simulink model "SemiOffline_Preprocessing_SCG3D"  (R2019a)
settings: Solver=FixedStepDiscrete  StartTime=0.0  StopTime=2*sim_time  FixedStep=1/fs  MaxStep=1/fs  RelTol=1e-3
undefined symbols (not defined in the file): fdesignblkfcn, fs, gcbh, tot_samples
settings Model: Creator=rcord  LastModifiedBy=rcord
settings DataIOCC: ExternalInput=[t, x, y, z]  LoadExternalInput=on
settings DebuggingCC: UnderSpecifiedDimensionMsg=warning

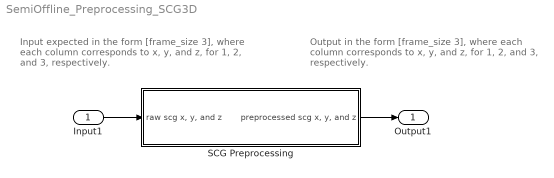
== system SemiOffline_Preprocessing_SCG3D ==
  note: Input expected in the form [frame_size 3],
      | where each column corresponds to x, y, and z,
      | for 1, 2, and 3, respectively.
  note: Output in the form [frame_size 3],
      | where each column corresponds to x, y, and z,
      | for 1, 2, and 3, respectively.
  Input1 : Inport  SampleTime=1/fs
  SCG Preprocessing : Subsystem  mask{param_scg_gain_mg=3333, param_scg_fc_lo=5, param_scg_fc_hi=40, param_scg_trans_bw=2.5}
      mask prompts: param_scg_gain_mg "V to mg Conversion Gain"; param_scg_fc_lo "Low Passband Frequency Corner (Hz)"; param_scg_fc_hi "High Passband Frequency Corner (Hz)"; param_scg_trans_bw "Transition bandwidth"
      mask init:
      | assignin('base','param_scg_gain_mg',param_scg_gain_mg)
      | assignin('base','param_scg_fc_lo',param_scg_fc_lo)
      | assignin('base','param_scg_fc_hi',param_scg_fc_hi)
      | assignin('base','param_scg_trans_bw',param_scg_trans_bw)
      mask DialogControl DescGroupVar Prompt: SCG Preprocessing
      mask DialogControl DescTextVar Prompt: The preprocesing of the three SCG x, y, and z components passed along a single signal input. The preprocessing consists of a amplifcaiton/conversion stage followed by a filtfilt operation (i.e. a front-back zero-phase FIR bandpass filter).
  Output1 : Outport
  wires:
  Input1/1 -> SCG Preprocessing/1("raw scg x, y, and z")
  SCG Preprocessing/1("preprocessed scg x, y, and z") -> Output1/1

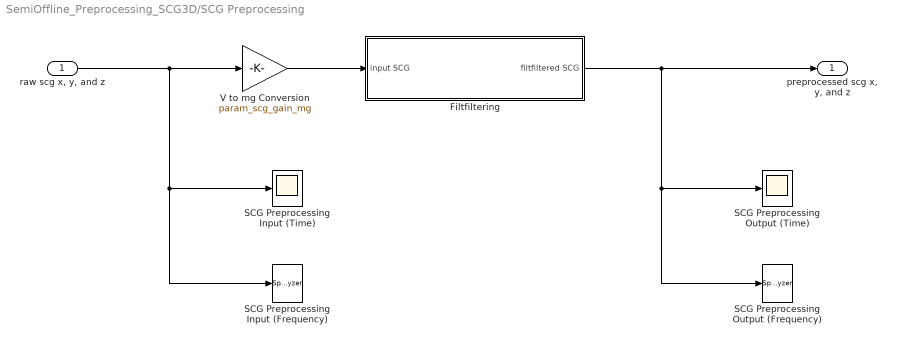
== system SemiOffline_Preprocessing_SCG3D/SCG Preprocessing ==
  "raw scg x, y, and z" : Inport
  Filtfiltering : Subsystem
  SCG Preprocessing Input (Frequency) : SpectrumAnalyzer
  SCG Preprocessing Input (Time) : Scope
  SCG Preprocessing Output (Frequency) : SpectrumAnalyzer
  SCG Preprocessing Output (Time) : Scope
  V to mg Conversion : Gain  Gain=param_scg_gain_mg
  "preprocessed scg x, y, and z" : Outport
  wires:
  V to mg Conversion/1 -> Filtfiltering/1(" input SCG")
  Filtfiltering/1(filtfiltered SCG) -> "preprocessed scg x, y, and z"/1, SCG Preprocessing Output (Frequency)/1, SCG Preprocessing Output (Time)/1
  "raw scg x, y, and z"/1 -> V to mg Conversion/1, SCG Preprocessing Input (Frequency)/1, SCG Preprocessing Input (Time)/1

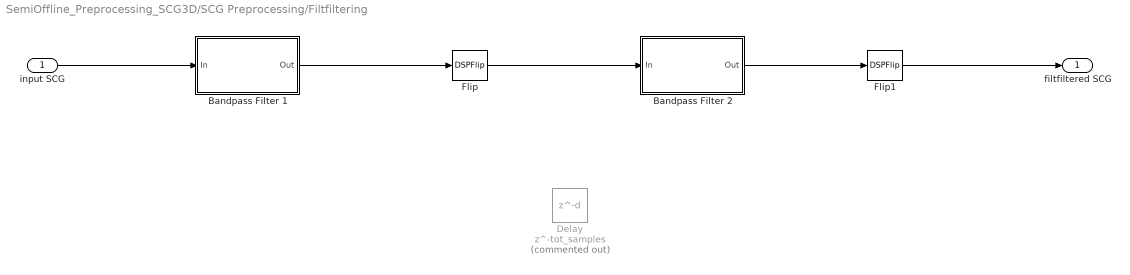
== system SemiOffline_Preprocessing_SCG3D/SCG Preprocessing/Filtfiltering ==
  " input SCG" : Inport
  Bandpass Filter 1 : Subsystem  DialogController=fdesignblkfcn  InitFcn=fdesignblkfcn(gcbh, {'InitFcn'});  mask(Bandpass Filter){}
      mask help: Design a bandpass filter
      settings: CopyFcn=fdesignblkfcn(gcbh, {'CopyFcn'});
      mask Help: helpview(mapfilelocation('dsp'), 'dspbandpassfilter');
      mask Display: disp('Bandpass');
  Bandpass Filter 2 : Subsystem  DialogController=fdesignblkfcn  InitFcn=fdesignblkfcn(gcbh, {'InitFcn'});  mask(Bandpass Filter){}
      mask help: Design a bandpass filter
      settings: CopyFcn=fdesignblkfcn(gcbh, {'CopyFcn'});
      mask Help: helpview(mapfilelocation('dsp'), 'dspbandpassfilter');
      mask Display: disp('Bandpass');
  Delay : Delay  Commented=on  DelayLength=tot_samples
  Flip : DSPFlip
  Flip1 : DSPFlip
  filtfiltered SCG : Outport
  wires:
  Bandpass Filter 2/1(Out) -> Flip1/1
  Bandpass Filter 1/1(Out) -> Flip/1
  Flip1/1 -> filtfiltered SCG/1
  " input SCG"/1 -> Bandpass Filter 1/1(In)
  Flip/1 -> Bandpass Filter 2/1(In)

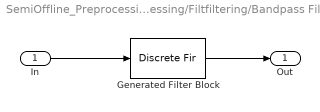
== system SemiOffline_Preprocessing_SCG3D/SCG Preprocessing/Filtfiltering/Bandpass Filter 1 ==
  In : Inport
  Generated Filter Block : DiscreteFir  Tag=BlockMethodSubSystem  Coefficients=[-0.000644776881089011221 -0.000343554860043022352 -0.000418089254709499275 -0.000488742609981019163 -0.000551243345798582566 -0.000600235305924576648 -0.00063171306769246806 -0.000640836865515264807 -0.000623577399542782373 -0.000575229334500284694 -0.000494985950960804763 -0.000381627044804629134 -0.000233865006442936121 -5.56678921839550995e-05 0.000150944750294620727 0.000380332853480295433 0.00062653849699591019 0.000881816649475024436 0.00113740319574445639 0.00138431406995232105 0.00161321911397308633 0.0018146043144366829 0.00198008854337072566 0.00210262259699513969 0.00217572124608666432 0.00219597055848480376 0.00216075573049529434 0.00207097175527305938 0.00192865213177504605 0.00173898123537951027 0.00150863042848189965 0.00124677018487260151 0.000963043907161496653 0.000669179660023357689 0.000376320878595885961 9.62462280283141939e-05 -0.000160563804743702409 -0.000384391646009586794 -0.000567507973019773342 -0.000704030812785294492 -0.00079079232930282504 -0.000826637258703924243 -0.000813548141499978168 -0.000755551211624549946 -0.000659215605623974577 -0.000532703240683185986 -0.000385888389387102669 -0.000229155313949030114 -7.35784921629424322e-05 7.06945997310475362e-05 0.000193741453659791903 0.000287790719150024911 0.000346383593154441817 0.000365847560832936172 0.000344383008930271859 0.000283347463518772609 0.000185853244975725074 5.79335170000474034e-05 -9.32933989238659894e-05 -0.000258576563413746212 -0.0004284890942197088 -0.000592821858813498285 -0.000742242260932749745 -0.00086783910074455324 -0.000962759059241456673 -0.0010215146506733989 -0.00104142267039370319 -0.00102169614249135237 -0.000964510497639283534 -0.000873959783460330681 -0.000756582912594168204 -0.000620183712708287848 -0.000474201473147084441 -0.000328149776762294532 -0.000192029162020909033 -7.46952916294248755e-05 1.57079301373542948e-05 7.32427637147023197e-05 9.36173902064841982e-05 7.54005127585129936e-05 1.91161807097391763e-05 -7.16595904837144548e-05 -0.000191710326143970493 -0.000333326478420456083 -0.000487918818970811197 -0.000645475596531724797 -0.000796262938914105698 -0.000930417408673228402 -0.0010396156115845801 -0.00111654678736693505 -0.00115650619497951069 -0.00115662609648395213 -0.00111707780801223997 -0.00104015953461484211 -0.000931040340278774074 -0.000796577490100713621 -0.000645746267254139169 -0.000488196428482681939 -0.000334541919957035403 -0.000194753410450029471 -7.83949421000261601e-05 6.83354906831558796e-06 5.48102364234399875e-05 6.22366935722899512e-05 2.80056891788165547e-05 -4.57953631900057979e-05 -0.000154930784782747748 -0.000292305286820631997 -0.000449364913192355558 -0.000615713486995709647 -0.000780661745517044676 -0.000933031005179838727 -0.0010628070138965556 -0.00116084839104745735 -0.00122045594744212178 -0.00123689017731540502 -0.0012086305976936663 -0.0011366220726097213 -0.00102507863635119484 -0.000880435884838085664 -0.000711770626707669291 -0.000529391845676479515 -0.00034502623282510952 -0.000170242786044573046 -1.64810979591180785e-05 0.000106463703824997253 0.000190367848146880136 0.000229854166427127706 0.000222059182005315641 0.000167606062212376521 6.98223655175191213e-05 -6.46609165418749691e-05 -0.000227063302337504646 -0.000406262186824843418 -0.000590230944417701126 -0.000766074161657273774 -0.000921613959220814486 -0.00104542488275643965 -0.00112839809981801569 -0.00116355855800205198 -0.00114734056156514806 -0.00107911583754525284 -0.000962004175138825779 -0.000801990744713897141 -0.000608297123417612983 -0.000392092411578965976 -0.000166510717696855047 5.49090292653681361e-05 0.000258408604381921798 0.000431569022470128867 0.000563523486343455978 0.000646306107611778783 0.000674792216429977577 0.000647704832457918168 0.000567118636300042089 0.00043900028457117998 0.000272243326566881476 7.87297422543196783e-05 -0.000127994233223484397 -0.000333009490540980173 -0.000521581473200367473 -0.000679514828449278999 -0.000794723347056151721 -0.000857432520348350765 ...(+15268 chars)]  InputProcessing=Columns as channels (frame based)
  Out : Outport
  wires:
  Generated Filter Block/1 -> Out/1
  In/1 -> Generated Filter Block/1

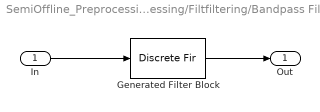
== system SemiOffline_Preprocessing_SCG3D/SCG Preprocessing/Filtfiltering/Bandpass Filter 2 ==
  In : Inport
  Generated Filter Block : DiscreteFir  Tag=BlockMethodSubSystem  Coefficients=[-0.000644776881089011221 -0.000343554860043022352 -0.000418089254709499275 -0.000488742609981019163 -0.000551243345798582566 -0.000600235305924576648 -0.00063171306769246806 -0.000640836865515264807 -0.000623577399542782373 -0.000575229334500284694 -0.000494985950960804763 -0.000381627044804629134 -0.000233865006442936121 -5.56678921839550995e-05 0.000150944750294620727 0.000380332853480295433 0.00062653849699591019 0.000881816649475024436 0.00113740319574445639 0.00138431406995232105 0.00161321911397308633 0.0018146043144366829 0.00198008854337072566 0.00210262259699513969 0.00217572124608666432 0.00219597055848480376 0.00216075573049529434 0.00207097175527305938 0.00192865213177504605 0.00173898123537951027 0.00150863042848189965 0.00124677018487260151 0.000963043907161496653 0.000669179660023357689 0.000376320878595885961 9.62462280283141939e-05 -0.000160563804743702409 -0.000384391646009586794 -0.000567507973019773342 -0.000704030812785294492 -0.00079079232930282504 -0.000826637258703924243 -0.000813548141499978168 -0.000755551211624549946 -0.000659215605623974577 -0.000532703240683185986 -0.000385888389387102669 -0.000229155313949030114 -7.35784921629424322e-05 7.06945997310475362e-05 0.000193741453659791903 0.000287790719150024911 0.000346383593154441817 0.000365847560832936172 0.000344383008930271859 0.000283347463518772609 0.000185853244975725074 5.79335170000474034e-05 -9.32933989238659894e-05 -0.000258576563413746212 -0.0004284890942197088 -0.000592821858813498285 -0.000742242260932749745 -0.00086783910074455324 -0.000962759059241456673 -0.0010215146506733989 -0.00104142267039370319 -0.00102169614249135237 -0.000964510497639283534 -0.000873959783460330681 -0.000756582912594168204 -0.000620183712708287848 -0.000474201473147084441 -0.000328149776762294532 -0.000192029162020909033 -7.46952916294248755e-05 1.57079301373542948e-05 7.32427637147023197e-05 9.36173902064841982e-05 7.54005127585129936e-05 1.91161807097391763e-05 -7.16595904837144548e-05 -0.000191710326143970493 -0.000333326478420456083 -0.000487918818970811197 -0.000645475596531724797 -0.000796262938914105698 -0.000930417408673228402 -0.0010396156115845801 -0.00111654678736693505 -0.00115650619497951069 -0.00115662609648395213 -0.00111707780801223997 -0.00104015953461484211 -0.000931040340278774074 -0.000796577490100713621 -0.000645746267254139169 -0.000488196428482681939 -0.000334541919957035403 -0.000194753410450029471 -7.83949421000261601e-05 6.83354906831558796e-06 5.48102364234399875e-05 6.22366935722899512e-05 2.80056891788165547e-05 -4.57953631900057979e-05 -0.000154930784782747748 -0.000292305286820631997 -0.000449364913192355558 -0.000615713486995709647 -0.000780661745517044676 -0.000933031005179838727 -0.0010628070138965556 -0.00116084839104745735 -0.00122045594744212178 -0.00123689017731540502 -0.0012086305976936663 -0.0011366220726097213 -0.00102507863635119484 -0.000880435884838085664 -0.000711770626707669291 -0.000529391845676479515 -0.00034502623282510952 -0.000170242786044573046 -1.64810979591180785e-05 0.000106463703824997253 0.000190367848146880136 0.000229854166427127706 0.000222059182005315641 0.000167606062212376521 6.98223655175191213e-05 -6.46609165418749691e-05 -0.000227063302337504646 -0.000406262186824843418 -0.000590230944417701126 -0.000766074161657273774 -0.000921613959220814486 -0.00104542488275643965 -0.00112839809981801569 -0.00116355855800205198 -0.00114734056156514806 -0.00107911583754525284 -0.000962004175138825779 -0.000801990744713897141 -0.000608297123417612983 -0.000392092411578965976 -0.000166510717696855047 5.49090292653681361e-05 0.000258408604381921798 0.000431569022470128867 0.000563523486343455978 0.000646306107611778783 0.000674792216429977577 0.000647704832457918168 0.000567118636300042089 0.00043900028457117998 0.000272243326566881476 7.87297422543196783e-05 -0.000127994233223484397 -0.000333009490540980173 -0.000521581473200367473 -0.000679514828449278999 -0.000794723347056151721 -0.000857432520348350765 ...(+15268 chars)]  InputProcessing=Columns as channels (frame based)
  Out : Outport
  wires:
  In/1 -> Generated Filter Block/1
  Generated Filter Block/1 -> Out/1
